simulink model "Simulaciontarea1"  (R2020b)
settings: Solver=VariableStepAuto  StartTime=0.0  StopTime=10.0  RelTol=1e-3
settings Model: Creator=maria  LastModifiedBy=maria

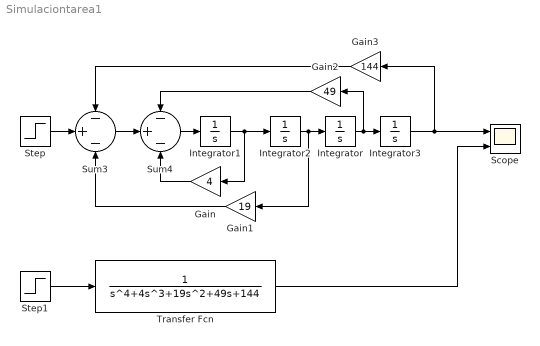
== system Simulaciontarea1 ==
  Gain : Gain  Gain=4
  Gain1 : Gain  Gain=19
  Gain2 : Gain  Gain=49
  Gain3 : Gain  Gain=144
  Integrator{,1..3} (4 alike) : Integrator
  Scope : Scope  NumInputPorts=2
  Step : Step  SampleTime=0
  Step1 : Step  SampleTime=0
  Sum3 : Sum  Inputs=-+-
  Sum4 : Sum  Inputs=-+-
  Transfer Fcn : TransferFcn  Denominator=[1 4 19 49 144]
  wires:
  Gain1/1 -> Sum3/3
  Sum3/1 -> Sum4/2
  Sum4/1 -> Integrator1/1
  Gain/1 -> Sum4/3
  Integrator1/1 -> Gain/1, Integrator2/1
  Integrator2/1 -> Gain1/1, Integrator/1
  Integrator/1 -> Gain2/1, Integrator3/1
  Gain2/1 -> Sum4/1
  Gain3/1 -> Sum3/1
  Integrator3/1 -> Gain3/1, Scope/1
  Step/1 -> Sum3/2
  Step1/1 -> Transfer Fcn/1
  Transfer Fcn/1 -> Scope/2
